simulink model "vers01"  (R2018a)
settings: Solver=VariableStepAuto  StartTime=0.0  StopTime=10.0  RelTol=1e-3
model workspace (MAT data in the model file):
  CONVERTER_DATA = [0  137.465208994  2.232; 0.1  137.065019157  2.075; 0.2  135.864449646  1.975; 0.3  135.664354728  1.846; 0.4  137.565256453  1.72; 0.5  140.366585312  1.564; 0.6  145.268910814  1.409; 0.7  152.872517717  1.254; 0.8  162.9773111  1.096; 0.81  164.27792807  1.08; 0.82  166.178829795  1.061; 0.83  167.979684062  1.043; 0.84  170.080680706  1.028; 0.85  172.781962105  1.012; 0.86  175.383196045  1.002; 0.87  179.585189333  1.002; 0.88  183.587087703  1.001; 0.89  189.890077635  0.998; 0.9  197.693779455  0.999; 0.92  215.902417037  1.001; 0.94  244.515990379  1.002]
  DOWN_TABLE = [0  5  20  35; 0  5  20  35; 0  5  25  40; 0  5  30  50; 0  30  50  80; 0  30  50  80]
  DOWN_TH_BP = [0; 5; 40; 50; 90; 100]
  EMAP = [-40  -44  -49  -53  -57  -61  -65  -70  -74  -78  -82; 215  117  85  66  44  29  10  -2  -13  -22  -32; 245  208  178  148  122  104  85  66  48  33  18; 264  260  241  219  193  167  152  133  119  96  85; 264  279  282  275  260  238  223  208  189  171  152; 267  290  293  297  290  275  260  256  234  212  193; 267  297  305  305  305  301  293  282  267  249  226; 267  301  308  312  319  323  319  316  297  279  253; 267  301  312  319  327  327  327  327  312  293  267; 267  301  312  319  327  334  334  334  319  305  275]
  Iei = 0.0219914882836
  NE_VEC = [800 1200 1600 2000 2400 2800 3200 3600 4000 4400 4800]
  TH_VEC = [0; 20; 30; 40; 50; 60; 70; 80; 90; 100]
  TWAIT = 2
  UP_TABLE = [10  30  50  1000000; 10  30  50  1000000; 15  30  50  1000000; 23  41  60  1000000; 40  70  100  1000000; 40  70  100  1000000]
  UP_TH_BP = [0; 25; 35; 50; 90; 100]
  VEHICLE_DATA = [3.23; 40; 0.02; 1; 12.0941478573; 0]
undefined symbols (not defined in the file): sigbuilder_block
settings Model: DataTypeOverride=Double  Creator=oolonthegreat  LastModifiedBy=oolonthegreat
settings DataIOCC: SaveOutput=off  SignalLogging=off  DSMLogging=off  SaveTime=off

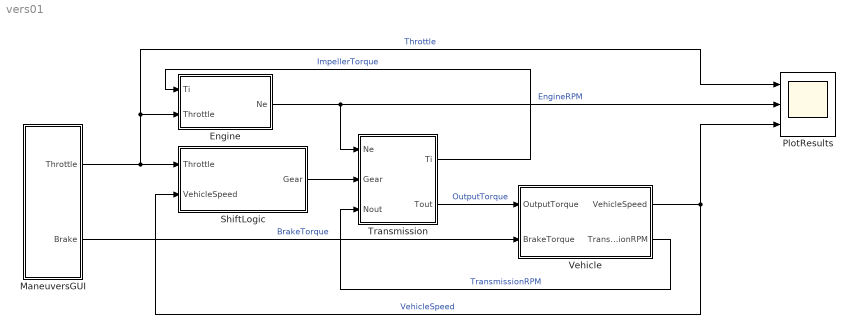
== system vers01 ==
  Engine : Subsystem
  ManeuversGUI : Subsystem  Tag=STV Subsys  LoadFcn=sigbuilder_block('load');  StartFcn=sigbuilder_block('start');  StopFcn=sigbuilder_block('stop');  ClipboardFcn=sigbuilder_block('clipboard');  mask(Sigbuilder block){tuvar=[0:10]}
      mask help: Sigbuilder GUI
      mask init:
      | tuvar = sigbuilder_block('maskInit');
      settings: CopyFcn=sigbuilder_block('copy');  DeleteFcn=sigbuilder_block('delete');  ModelCloseFcn=sigbuilder_block('modelClose');  PreSaveFcn=sigbuilder_block('preSave');  PauseFcn=sigbuilder_block('pause')  ContinueFcn=sigbuilder_block('continue')  NameChangeFcn=sigbuilder_block('namechange');  OpenFcn=sigbuilder_block('open',[80.8 328 413.6 257.6 ]);  CloseFcn=sigbuilder_block('close');
      mask Display: plot(0, 0, 100, 100,[2, 2, 32, 32, 2], [68, 8, 8, 68, 68],[32, 2], [38, 38], [32, 19, 2],[53, 60, 44], [32, 17, 17, 2],[16, 16, 31, 31]);txt = getActiveGroup(gcbh);text(2, 100, txt,'verticalAlignment', 'top');
  PlotResults : Scope  NumInputPorts=3
  ShiftLogic : Stateflow chart  TreatAsAtomicUnit=on
  Transmission : Subsystem
  Vehicle : Subsystem  mask(vehicle model){Rfd=VEHICLE_DATA(1), rload0=VEHICLE_DATA(2), rload2=VEHICLE_DATA(3), Rw=VEHICLE_DATA(4), Iv=VEHICLE_DATA(5), N20=VEHICLE_DATA(6)/VEHICLE_DATA(4)*VEHICLE_DATA(1)}
      mask prompts: Rfd "final drive ratio"; rload0 "drag friction at wheels"; rload2 "aerodynamic drag"; Rw "wheel radius"; Iv "vehicle inertia"; N20 "initial transmission output speed"
      mask help: vehicle dynamics: torque input from trans., outputs are input speed (transmission output) and vehicle speed
      mask Display: image([matlabroot,'/toolbox/simulink/simdemos/automotive/html/NSX_3Colors.jpg'])
  wires:
  ManeuversGUI/2(Brake) -> Vehicle/2(BrakeTorque)  "BrakeTorque"
  Vehicle/1(VehicleSpeed) -> ShiftLogic/2(VehicleSpeed), PlotResults/3  "VehicleSpeed"
  ShiftLogic/1(Gear) -> Transmission/2(Gear)
  Transmission/2(Tout) -> Vehicle/1(OutputTorque)  "OutputTorque"
  Transmission/1(Ti) -> Engine/1(Ti)  "ImpellerTorque"
  Engine/1(Ne) -> Transmission/1(Ne), PlotResults/2  "EngineRPM"
  Vehicle/2(TransmissionRPM) -> Transmission/3(Nout)  "TransmissionRPM"
  ManeuversGUI/1(Throttle) -> Engine/2(Throttle), PlotResults/1, ShiftLogic/1(Throttle)  "Throttle"

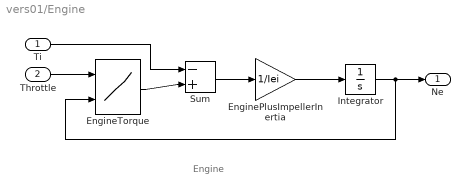
== system vers01/Engine ==
  note: Engine
  Ti : Inport  Unit=ft*lbf@torque
  Throttle : Inport  Port=2  Unit=%
  EnginePlusImpellerInertia : Gain  Gain=1/Iei  SaturateOnIntegerOverflow=on  OutDataTypeStr=Inherit: Same as input  ParamDataTypeStr=Inherit: Same as input
  EngineTorque : Lookup_n-D  BreakpointsForDimension1=TH_VEC  BreakpointsForDimension2=NE_VEC  Table=EMAP  InputSameDT=on
  Integrator : Integrator  InitialCondition=1000  LimitOutput=on  UpperSaturationLimit=6000  LowerSaturationLimit=600  ZeroCross=off
  Sum : Sum  Inputs=-+  SaturateOnIntegerOverflow=on  InputSameDT=on  OutDataTypeStr=Inherit: Same as first input
  Ne : Outport  Unit=rpm
  wires:
  Ti/1 -> Sum/1
  Throttle/1 -> EngineTorque/1
  Integrator/1 -> EngineTorque/2, Ne/1
  Sum/1 -> EnginePlusImpellerInertia/1
  EnginePlusImpellerInertia/1 -> Integrator/1
  EngineTorque/1 -> Sum/2

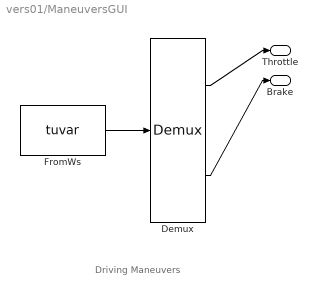
== system vers01/ManeuversGUI ==
  note: Driving Maneuvers
  Demux : Demux  Tag=STV Demux  Outputs=2
  FromWs : FromWorkspace  Tag=STV FromWs  VariableName=tuvar  SampleTime=0
      SigBuilderData=|
      | dataSet(1).timeRange = [0 50]
      | dataSet(1).name = 'Passing Maneuver'
      | dataSet(2).timeRange = [0 50]
      | dataSet(2).name = 'Gradual Acceleration'
      | dataSet(3).timeRange = [0 50]
      | dataSet(3).name = 'Hard braking'
      | dataSet(4).timeRange = [0 50]
      | dataSet(4).name = 'Coasting'
      | sbobj.Groups(1).Name = 'Passing Maneuver'
      | sbobj.Groups(1).Signals(1).Name = 'Throttle'
      | sbobj.Groups(1).Signals(1).XData = [0 14.9 15 50]
      | sbobj.Groups(1).Signals(1).YData = [60 40 100 58.8235294118]
      | sbobj.Groups(1).Signals(2).Name = 'Brake'
      | sbobj.Groups(1).Signals(2).XData = [0 50]
      | sbobj.Groups(1).Signals(2).YData = [0 0]
      | sbobj.Groups(2).Name = 'Gradual Acceleration'
      | sbobj.Groups(2).Signals(1).Name = 'Throttle'
      | sbobj.Groups(2).Signals(1).XData = [0 50]
      | sbobj.Groups(2).Signals(1).YData = [13.4 24]
      | sbobj.Groups(2).Signals(2).Name = 'Brake'
      | sbobj.Groups(2).Signals(2).XData = [0 50]
      | sbobj.Groups(2).Signals(2).YData = [0 0]
      | sbobj.Groups(3).Name = 'Hard braking'
      | sbobj.Groups(3).Signals(1).Name = 'Throttle'
      | sbobj.Groups(3).Signals(1).XData = [0 5.1 5.1 50]
      | sbobj.Groups(3).Signals(1).YData = [50 50 1 1]
      | sbobj.Groups(3).Signals(2).Name = 'Brake'
      | sbobj.Groups(3).Signals(2).XData = [0 10 10 50]
      | sbobj.Groups(3).Signals(2).YData = [0 0 325 325]
      | sbobj.Groups(4).Name = 'Coasting'
      | sbobj.Groups(4).Signals(1).Name = 'Throttle'
      | sbobj.Groups(4).Signals(1).XData = [0 4.8 4.8 50]
      | sbobj.Groups(4).Signals(1).YData = [80 80 1 1]
      | sbobj.Groups(4).Signals(2).Name = 'Brake'
      | sbobj.Groups(4).Signals(2).XData = [0 50]
      | sbobj.Groups(4).Signals(2).YData = [0 0]
  Throttle : Outport  Tag=STV Outport
  Brake : Outport  Tag=STV Outport  Port=2
  wires:
  FromWs/1 -> Demux/1
  Demux/1 -> Throttle/1
  Demux/2 -> Brake/1

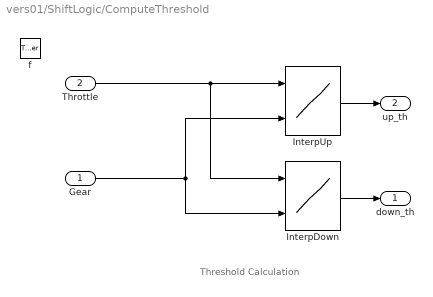
== system vers01/ShiftLogic/ComputeThreshold ==
  note: Threshold Calculation
  Gear : Inport
  Throttle : Inport  Port=2
  f : TriggerPort  TriggerType=function-call  VariantControl=(inherit)
      settings: CopyFcn=Stateflow.SLINSF.SimulinkMan.removeBlockPreDeleteFcn  PreDeleteFcn=Stateflow.SLINSF.SimulinkMan.unsafePredeleteFcn
  InterpDown : Lookup_n-D  BreakpointsForDimension1=DOWN_TH_BP  BreakpointsForDimension2=[1:4]  Table=DOWN_TABLE  OutDataTypeStr=double  LockScale=on
  InterpUp : Lookup_n-D  BreakpointsForDimension1=UP_TH_BP  BreakpointsForDimension2=[1:4]  Table=UP_TABLE  OutDataTypeStr=double  LockScale=on
  down_th : Outport  InitialOutput=0
  up_th : Outport  Port=2  InitialOutput=0
  wires:
  InterpUp/1 -> up_th/1
  InterpDown/1 -> down_th/1
  Throttle/1 -> InterpDown/1, InterpUp/1
  Gear/1 -> InterpDown/2, InterpUp/2

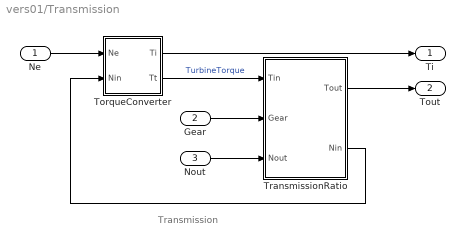
== system vers01/Transmission ==
  note: Transmission
  Ne : Inport  Unit=rpm
  Gear : Inport  Port=2  Unit=1
  Nout : Inport  Port=3  Unit=rpm
  TorqueConverter : Subsystem  mask(torque converter){speedratio=CONVERTER_DATA(:,1), Kfactor=CONVERTER_DATA(:,2), Torkratio=CONVERTER_DATA(:,3)}
      mask prompts: speedratio "speed ratio"; Kfactor "K factor"; Torkratio "torque ratio"
      mask help: torque converter
      mask Help: Torque converter input and output torques are computed as a function of the input and output speeds
      mask Display: plot([cos([90:10:450]*pi/180),.63*cos([90:10:450]*pi/180),.63*cos([90:10:240]*pi/180),cos([240:10:300]*pi/180),.63*cos([300]*pi/180)],[sin([90:10:450]*pi/180),.63*sin([90:10:450]*pi/180)+.1,.63*sin([90:10:240]*pi/180)+.1,sin([240:10:300]*pi/180),.63*sin([300]*pi/180)+.1])
  TransmissionRatio : Subsystem
  Ti : Outport  Unit=ft*lbf@torque
  Tout : Outport  Port=2  Unit=ft*lbf@torque
  wires:
  TransmissionRatio/1(Tout) -> Tout/1
  TorqueConverter/1(Ti) -> Ti/1
  Nout/1 -> TransmissionRatio/3(Nout)
  Gear/1 -> TransmissionRatio/2(Gear)
  Ne/1 -> TorqueConverter/1(Ne)
  TransmissionRatio/2(Nin) -> TorqueConverter/2(Nin)
  TorqueConverter/2(Tt) -> TransmissionRatio/1(Tin)  "TurbineTorque"

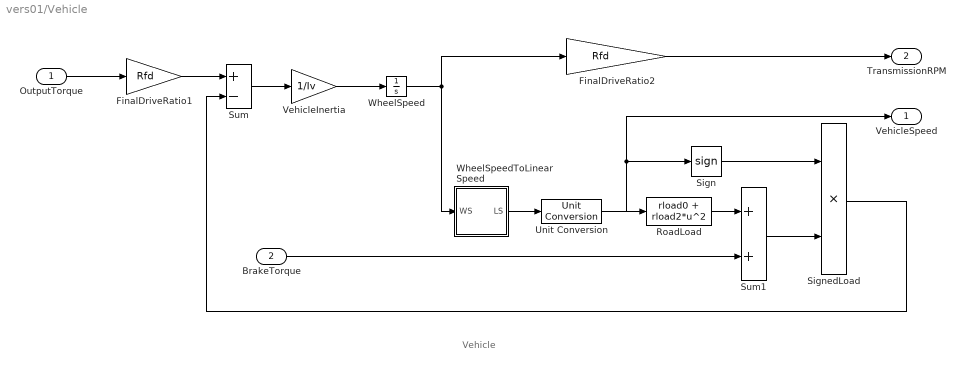
== system vers01/Vehicle ==
  note: Vehicle
  OutputTorque : Inport  Unit=ft*lbf@torque
  BrakeTorque : Inport  Port=2  Unit=ft*lbf@torque
  FinalDriveRatio1 : Gain  Gain=Rfd  SaturateOnIntegerOverflow=on  OutDataTypeStr=Inherit: Same as input  ParamDataTypeStr=Inherit: Same as input
  FinalDriveRatio2 : Gain  Gain=Rfd  SaturateOnIntegerOverflow=on  OutDataTypeStr=Inherit: Same as input  ParamDataTypeStr=Inherit: Same as input
  RoadLoad : Fcn  Expr=rload0 + rload2*u^2
  Sign : Signum
  SignedLoad : Product  SaturateOnIntegerOverflow=on  InputSameDT=on  OutDataTypeStr=Inherit: Same as first input
  Sum : Sum  Inputs=+-  SaturateOnIntegerOverflow=on  InputSameDT=on  OutDataTypeStr=Inherit: Same as first input
  Sum1 : Sum  SaturateOnIntegerOverflow=on  InputSameDT=on  OutDataTypeStr=Inherit: Same as first input
  Unit Conversion : UnitConversion
  VehicleInertia : Gain  Gain=1/Iv  SaturateOnIntegerOverflow=on  OutDataTypeStr=Inherit: Same as input  ParamDataTypeStr=Inherit: Same as input
  WheelSpeed : Integrator  InitialCondition=N20/Rfd  ZeroCross=off
  WheelSpeedToLinearSpeed : Subsystem
  VehicleSpeed : Outport  Unit=mph
  TransmissionRPM : Outport  Port=2  Unit=rpm
  wires:
  FinalDriveRatio2/1 -> TransmissionRPM/1
  BrakeTorque/1 -> Sum1/2
  Sum1/1 -> SignedLoad/2
  RoadLoad/1 -> Sum1/1
  Sign/1 -> SignedLoad/1
  SignedLoad/1 -> Sum/2
  OutputTorque/1 -> FinalDriveRatio1/1
  VehicleInertia/1 -> WheelSpeed/1
  Sum/1 -> VehicleInertia/1
  Unit Conversion/1 -> VehicleSpeed/1, Sign/1, RoadLoad/1
  WheelSpeed/1 -> WheelSpeedToLinearSpeed/1(WS), FinalDriveRatio2/1
  FinalDriveRatio1/1 -> Sum/1
  WheelSpeedToLinearSpeed/1(LS) -> Unit Conversion/1

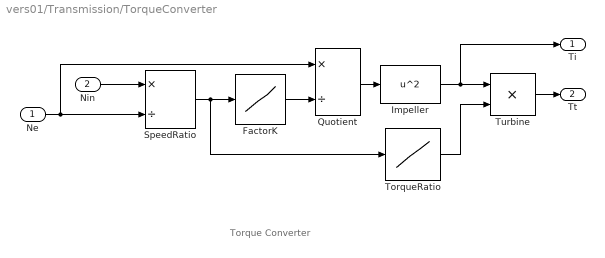
== system vers01/Transmission/TorqueConverter ==
  note: Torque Converter
  Ne : Inport
  Nin : Inport  Port=2
  FactorK : Lookup_n-D  NumberOfTableDimensions=1  BreakpointsForDimension1=speedratio  Table=Kfactor  SaturateOnIntegerOverflow=on  InputSameDT=on
  Impeller : Fcn  Expr=u^2
  Quotient : Product  Inputs=*/  SaturateOnIntegerOverflow=on  InputSameDT=on  OutDataTypeStr=Inherit: Same as first input
  SpeedRatio : Product  Inputs=*/  SaturateOnIntegerOverflow=on  InputSameDT=on  OutDataTypeStr=Inherit: Same as first input
  TorqueRatio : Lookup_n-D  NumberOfTableDimensions=1  BreakpointsForDimension1=speedratio  Table=Torkratio  SaturateOnIntegerOverflow=on  InputSameDT=on
  Turbine : Product  SaturateOnIntegerOverflow=on  InputSameDT=on  OutDataTypeStr=Inherit: Same as first input
  Ti : Outport
  Tt : Outport  Port=2
  wires:
  TorqueRatio/1 -> Turbine/2
  Quotient/1 -> Impeller/1
  FactorK/1 -> Quotient/2
  SpeedRatio/1 -> TorqueRatio/1, FactorK/1
  Impeller/1 -> Turbine/1, Ti/1
  Turbine/1 -> Tt/1
  Ne/1 -> SpeedRatio/2, Quotient/1
  Nin/1 -> SpeedRatio/1

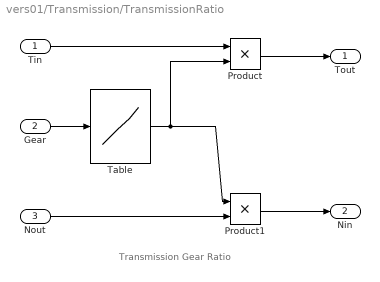
== system vers01/Transmission/TransmissionRatio ==
  note: Transmission Gear Ratio
  Tin : Inport  Unit=ft*lbf@torque
  Gear : Inport  Port=2  Unit=1
  Nout : Inport  Port=3  Unit=rpm
  Product : Product  SaturateOnIntegerOverflow=on  InputSameDT=on  OutDataTypeStr=Inherit: Same as first input
  Product1 : Product  SaturateOnIntegerOverflow=on  InputSameDT=on  OutDataTypeStr=Inherit: Same as first input
  Table : Lookup_n-D  NumberOfTableDimensions=1  BreakpointsForDimension1=[1 2 3 4]  Table=[2.393 1.450 1.000 0.677]  OutDataTypeStr=double  SaturateOnIntegerOverflow=on  InputSameDT=on  LockScale=on
  Tout : Outport  Unit=ft*lbf@torque
  Nin : Outport  Port=2  Unit=rpm
  wires:
  Table/1 -> Product1/1, Product/2
  Nout/1 -> Product1/2
  Product1/1 -> Nin/1
  Product/1 -> Tout/1
  Tin/1 -> Product/1
  Gear/1 -> Table/1

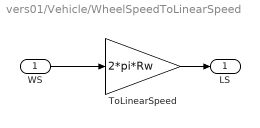
== system vers01/Vehicle/WheelSpeedToLinearSpeed ==
  WS : Inport  Unit=rpm
  ToLinearSpeed : Gain  Gain=2*pi*Rw  SaturateOnIntegerOverflow=on  OutDataTypeStr=Inherit: Same as input  ParamDataTypeStr=Inherit: Same as input
  LS : Outport  Unit=ft/min
  wires:
  ToLinearSpeed/1 -> LS/1
  WS/1 -> ToLinearSpeed/1

== stateflow chart vers01/ShiftLogic ==
  settings: updateMethod=DISCRETE  sampleTime=0.04
  state gear_state [parallel]
    settings: executionOrder=1
    state first
      entry:
      Gear = 1;
    state second
      entry:
      Gear = 2;
    state third
      entry:
      Gear = 3;
    state fourth
      entry:
      Gear = 4;
    (default) -> first
    second -> third [order 1] : UP
    first -> second : UP
    third -> fourth [order 1] : UP
    third -> second [order 2] : DOWN
    second -> first [order 2] : DOWN
    fourth -> third : DOWN
  state selection_state [parallel]
    during:
    [down_th, up_th] = ComputeThreshold(Gear,Throttle);
    settings: executionOrder=2
    state steady_state
    state upshifting
    state downshifting
    (default) -> steady_state
    steady_state -> upshifting [order 1] : [VehicleSpeed > up_th]
    steady_state -> downshifting [order 2] : [VehicleSpeed < down_th]
    downshifting -> steady_state [order 1] : after(TWAIT,tick)
        | [VehicleSpeed <= down_th]
        | {gear_state.DOWN}
    downshifting -> steady_state [order 2] : [VehicleSpeed > down_th]
    upshifting -> steady_state [order 1] : after(TWAIT,tick)
        | [VehicleSpeed >= up_th]
        | {gear_state.UP}
    upshifting -> steady_state [order 2] : [VehicleSpeed < up_th]
  state [down_th,up_th] = ComputeThreshold(Gear,Throttle) [function]
  data: Gear function_input; Throttle function_input; down_th function_output; up_th function_output; Throttle input double; VehicleSpeed input double; Gear output fixdt(0,8,5) [1..4]; TWAIT parameter fixdt(0,8,6); down_th local double; up_th local double
  events: DOWN local EITHER_EDGE_EVENT; UP local EITHER_EDGE_EVENT
